simulink model "simulink_function"  (R2014b)
settings: Solver=ode45  StartTime=0.0  StopTime=10.0  RelTol=1e-3
settings Model: Creator=tkr5kor  LastModifiedBy=tkr5kor

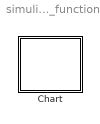
== system simulink_function ==
  Chart : Stateflow chart  TreatAsAtomicUnit=on

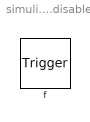
== system simulink_function/Chart/state.disable ==
  f : TriggerPort  TriggerType=function-call
      settings: CopyFcn=Stateflow.SLINSF.SimulinkMan.removeBlockPreDeleteFcn  PreDeleteFcn=Stateflow.SLINSF.SimulinkMan.unsafePredeleteFcn

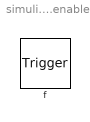
== system simulink_function/Chart/state.enable ==
  f : TriggerPort  TriggerType=function-call
      settings: CopyFcn=Stateflow.SLINSF.SimulinkMan.removeBlockPreDeleteFcn  PreDeleteFcn=Stateflow.SLINSF.SimulinkMan.unsafePredeleteFcn

== stateflow chart simulink_function/Chart ==
  state state
    state state2
    state enable [function]
    state disable [function]
